simulink model "S3"  (R2023b)
settings: Solver=FixedStepAuto  StartTime=0.0  StopTime=10  FixedStep=Step_T  RelTol=1e-3
values from neighbouring files (symbols this model uses):
  Step_T = 0.001    [P_sim.m]
  x_1_0 = 0.2    [P_sim.m]
  x_2_0 = 0.5    [P_sim.m]
  x_3_0 = -1    [P_sim.m]
undefined symbols (not defined in the file or in its folder): pam
settings Model: Creator=admin  LastModifiedBy=admin

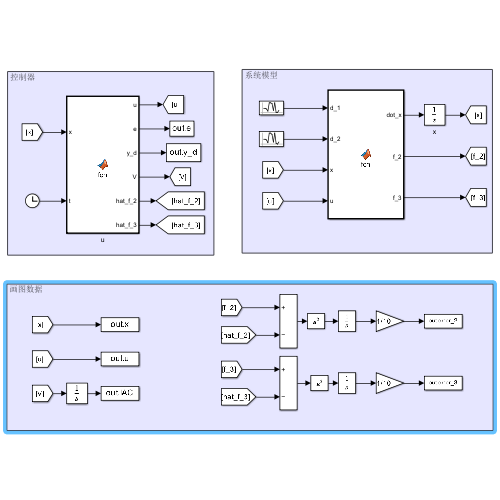
[thumbnail: Simulink's stored preview of the top-level diagram]
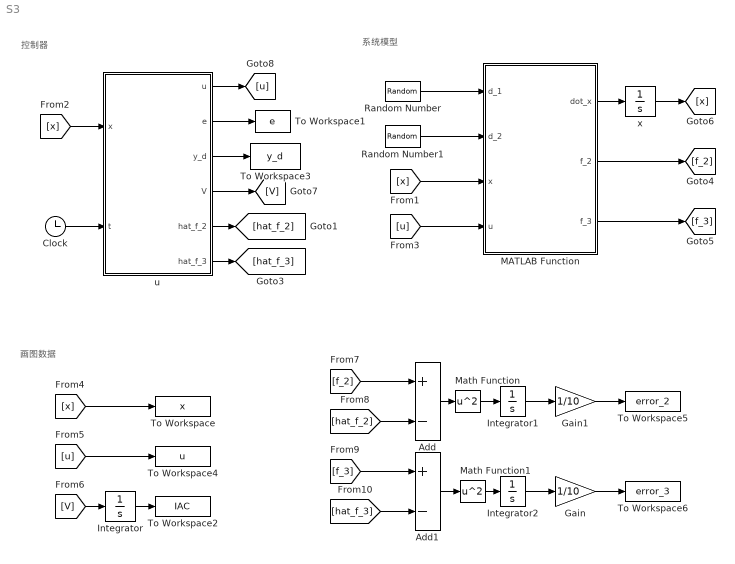
== system S3 ==
  note: 画图数据
  note: 系统模型
  note: 控制器
  Add : Sum  Inputs=+-
  Add1 : Sum  Inputs=+-
  Clock : Clock
  Gain : Gain  Gain=1/10
  Gain1 : Gain  Gain=1/10
  Integrator : Integrator
  Integrator1 : Integrator
  Integrator2 : Integrator
  MATLAB Function : MATLAB Function  TreatAsAtomicUnit=on
  Math Function : Math  Operator=square
  Math Function1 : Math  Operator=square
  Random Number : RandomNumber  Variance=pam.d*pam.d  Seed=-1  SampleTime=Step_T
  Random Number1 : RandomNumber  Variance=pam.d*pam.d  Seed=1  SampleTime=Step_T
  To Workspace : ToWorkspace  VariableName=x  SaveFormat=Timeseries  SampleTime=-1
  To Workspace1 : ToWorkspace  VariableName=e  SaveFormat=Timeseries  SampleTime=-1
  To Workspace2 : ToWorkspace  VariableName=IAC  SaveFormat=Timeseries  SampleTime=-1
  To Workspace3 : ToWorkspace  VariableName=y_d  SaveFormat=Timeseries  SampleTime=-1
  To Workspace4 : ToWorkspace  VariableName=u  SaveFormat=Timeseries  SampleTime=-1
  To Workspace5 : ToWorkspace  VariableName=error_2  SaveFormat=Timeseries  SampleTime=-1
  To Workspace6 : ToWorkspace  VariableName=error_3  SaveFormat=Timeseries  SampleTime=-1
  u : MATLAB Function  TreatAsAtomicUnit=on
  x : Integrator  InitialCondition=[x_1_0;x_2_0;x_3_0]
  wires:
  MATLAB Function/1(dot_x) -> x/1
  u/2(e) -> To Workspace1/1
  u/3(y_d) -> To Workspace3/1
  Clock/1 -> u/2(t)
  Random Number/1 -> MATLAB Function/1(d_1)
  Random Number1/1 -> MATLAB Function/2(d_2)
  u/5(hat_f_2) -> [hat_f_2]
  u/6(hat_f_3) -> [hat_f_3]
  MATLAB Function/2(f_2) -> [f_2]
  MATLAB Function/3(f_3) -> [f_3]
  x/1 -> [x]
  [x] -> MATLAB Function/3(x)
  [x] -> u/1(x)
  u/4(V) -> [V]
  u/1(u) -> [u]
  [u] -> MATLAB Function/4(u)
  [x] -> To Workspace/1
  [u] -> To Workspace4/1
  Integrator/1 -> To Workspace2/1
  [V] -> Integrator/1
  [f_2] -> Add/1
  [hat_f_2] -> Add/2
  Add/1 -> Math Function/1
  Integrator1/1 -> Gain1/1
  [f_3] -> Add1/1
  Add1/1 -> Math Function1/1
  Integrator2/1 -> Gain/1
  [hat_f_3] -> Add1/2
  Gain/1 -> To Workspace6/1
  Gain1/1 -> To Workspace5/1
  Math Function/1 -> Integrator1/1
  Math Function1/1 -> Integrator2/1

== matlab function S3/u ==
  data: x input; t input; u output; e output; pam parameter; y_d output; V output; hat_f_2 output; hat_f_3 output
function [u,e,y_d,V,hat_f_2,hat_f_3]  = fcn(x,t,pam)

y_d = sin(t);
dot_y_d = cos(t);
ddot_y_d = -sin(t);
dddot_y_d = -cos(t);

x_1 = x(1);
x_2 = x(2);
x_3 = x(3);

z_2 = [sin(x_1);x_2];
z_3 = [x_2;x_3];

dot_x_1 = x_2;
dot_x_2 = x_3+pam.hat_theta_2'*z_2;


pdot_alpha_2_x_1 = pam.hat_theta_2'*[cos(x_1);0]; 
pdot_alpha_2_x_2 = pam.hat_theta_2'*[0;1];

pdot_alpha_2_e_1 = -pam.lambda_1;

%% 第一阶
e_1 = x_1 - y_d;
alpha_1 = -pam.lambda_1*e_1+dot_y_d;
 
%% 第二阶
e_2 = x_2 - alpha_1;

dot_e_1 = dot_x_1-dot_y_d;
pdot_alpha_1_e_1 = -pam.lambda_1;
pdot_alpha_1_dy_d = 1;
dot_alpha_1 = pdot_alpha_1_e_1*dot_e_1+pdot_alpha_1_dy_d*ddot_y_d;

alpha_2 = -pam.lambda_2*e_2-pam.hat_theta_2'*z_2+dot_alpha_1;

%% 第三阶
e_3 = x_3 - alpha_2;

dot_e_2 = dot_x_2-dot_alpha_1;
pdot_alpha_2_e_1 = 0;
pdot_alpha_2_e_2 = -pam.lambda_2;
pdot_alpha_2_x_1 = -pam.hat_theta_2'*[cos(x_1);0]; 
pdot_alpha_2_x_2 = -pam.hat_theta_2'*[0;1]+pdot_alpha_1_e_1;
pdot_alpha_2_dy_d = -pdot_alpha_1_e_1;
pdot_alpha_2_ddy_d = pdot_alpha_1_dy_d;
dot_alpha_2 = pdot_alpha_2_e_1*dot_e_1+pdot_alpha_2_e_2*dot_e_2+pdot_alpha_2_x_1*dot_x_1+pdot_alpha_2_x_2*dot_x_2+pdot_alpha_2_dy_d*ddot_y_d+pdot_alpha_2_ddy_d*dddot_y_d;

u = -pam.lambda_3*e_3-pam.hat_theta_3'*z_3+dot_alpha_2;

e = [e_1;e_2;e_3];

V = e_1^2+u^2;

hat_f_2 = pam.hat_theta_2'*z_2;
hat_f_3 = pam.hat_theta_3'*z_3;

== matlab function S3/MATLAB Function ==
  data: d_1 input; d_2 input; x input; dot_x output; u input; pam parameter; f_2 output; f_3 output
function [dot_x,f_2,f_3]  = fcn(d_1,d_2,x,u,pam)

x_1 = x(1);
x_2 = x(2);
x_3 = x(3);

dot_x_1 = x_2;
dot_x_2 = x_3+pam.M/pam.D*sin(x_1)-pam.B/pam.D*x_2+d_1;
dot_x_3 = u+pam.K_m/pam.L*x_2-pam.J/pam.L*x_3+d_2;

dot_x = [dot_x_1;dot_x_2;dot_x_3];

f_2 = pam.M/pam.D*sin(x_1)-pam.B/pam.D*x_2;
f_3 = pam.K_m/pam.L*x_2-pam.J/pam.L*x_3;
